simulink model "LPDs_single_agent_tech"  (R2023b)
settings: Solver=VariableStepAuto  StartTime=0.0  StopTime=24  FixedStep=0.005  RelTol=1e-6
undefined symbols (not defined in the file): battery_capacity_state_lower_limit, battery_capacity_state_upper_limit, battery_charge_power_state_lower_limit, battery_charge_power_state_upper_limit, battery_discharge_power_state_lower_limit, battery_discharge_power_state_upper_limit, battery_initial_capacity, battery_SOC_state_lower_limit, battery_SOC_state_upper_limit, EV_load_priority_factor, EV_load_rating, EV_load_state_lower_limit, EV_load_state_upper_limit, micro_grid_controller_power_state_lower_limit, micro_grid_controller_power_state_upper_limit, nano_grid_controller_power_rating, nano_grid_controller_power_state_lower_limit, nano_grid_controller_power_state_upper_limit, PV_power_rating, PV_power_state_lower_limit, PV_power_state_upper_limit, static_load_priority_factor, static_load_rating, static_load_state_lower_limit, static_load_state_upper_limit, sum_power_threshold_lower_limit, sum_power_threshold_upper_limit, TCL_load_priority_factor, TCL_load_rating, TCL_load_state_lower_limit, TCL_load_state_upper_limit, Wind_power_rating, Wind_power_state_lower_limit, Wind_power_state_upper_limit
libraries: spsStairGeneratorLib x13, simulink x7, slpidlib x2, rllib x2
(part 2 of 4)

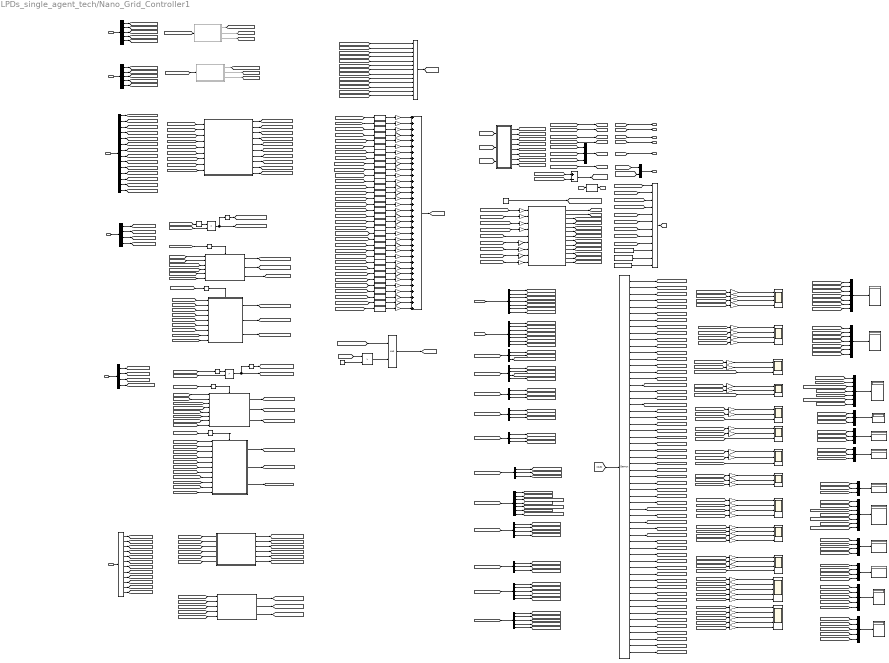
== system LPDs_single_agent_tech/Nano_Grid_Controller1 ==
  note: PV
  note: don't need I think so lets see it latter ???????????
  note: microgrid is least source
  note: nano grid is least priority source, its power usage will be punished:
      | if nanogrid is forecasting power supply
      | if nano grid is forecasting power consumption OR
      | if PV is NOT fully utilized OR
      | if wind is NOT fully utilized
  note: +ve = supply power
      | -ve = consume power
  note: Controller receiving
      | Information
      | ------------------------->
  note: Controller Transmitting
      | Information
  note: PV Power System parameters
      | ----------------------------------------------------------------------------------
  note: Wind
  note: BESS
  note: Load
  note: Observations / States / inputs
  note: Rewards / Punishments
  note: Battery is full and charging
      | than punish
  note: Micro Grid
  note: Nano Grid
  note: Wind Power System parameters
      | ----------------------------------------------------------------------------------
  note: Battery Power System parameters
      | ----------------------------------------------------------------------------------
  note: Nano Grid parameters
      | ----------------------------------------------------------------------------------
  note: Micro grid parameters
      | ----------------------------------------------------------------------------------
  note: Load parameters
      | ----------------------------------------------------------------------------------
  note: Power balance
      | ----------------------------------------------------------------------------------
  note: Nano Grid as source
      | ----------------------------------------------------------------------------------
  note: punish only if resources are not fully utilized
      | -10 points
  note: punish only if resources are not fully utilized
      | -10 points
  note: Battery Power -----> Battery Capacity (kWh) -----> Battery SOC Battery Charge Power
      | Battery Discharge Power
  PV1_input : Inport
  Wind_input : Inport  Port=2
  MG_Input : Inport  Port=3
  BESS_Input : Inport  Port=4
  Load_Input : Inport  Port=5
  NGC2_input : Inport  Port=6
  Abs1 : Abs  SaturateOnIntegerOverflow=off
  Abs2 : Abs  SaturateOnIntegerOverflow=off
  BESS : Subsystem
  Chart : Stateflow chart  TreatAsAtomicUnit=on
      settings: PortSchema="{\"entries\":[{\"content\":{\"sides\":[{\"content\":{\"connectorIds\":[\"In9\",\"In6\",\"In7\",\"In8\",\"In5\",\"In1\",\"In2\",\"In3\",\"In4\"]},\"type\":\"ConnectorPlacement.EquallySpacedRectSide\",\"uuid\":\"f3048845-fd52-425a-ab3b-550a9eb5c4bb\"},{\"content\":{\"connectorIds\":[\"Out1\",\"Out2\",\"Out3\",\"Out4\",\"Out10\",\"Out5\",\"Out6\",\"Out7\",\"Out9\",\"Out8\",\"Out11\",\"Out13\",\"Out12\"],\"side\":\"RIGHT\"},\"type\":\"ConnectorPlacement.EquallySpacedRectSide\",\"uuid\":\"2d1173df-378c-4293-a498-92c6385b9f9f\"},{\"content\":{\"side\":\"TOP\"},\"type\":\"ConnectorPlacement.EquallySpacedRectSide\",\"uuid\":\"05862f1f-9d24-4b39-880b-c5be5c8acb5d\"}]},\"type\":\"ConnectorPlacement.EquallySpacedConnector\",\"uuid\":\"30ceb18a-58fc-4555-bcd7-9edbd3426fbd\"}],\"packageUris\":[\"http://schema.mathworks.com/mf0/Connector/R2020b\"],\"version\":\"1.0\"}"
  Constant : Constant  Value=50
  Constant18 : Constant  Value=TCL_load_priority_factor
  Constant19 : Constant  Value=EV_load_priority_factor
  Constant20 : Constant  Value=static_load_priority_factor
  Constant6 : Constant  Value=0.95
  Data Type Conversion{10,12,14..45} (34 alike) : DataTypeConversion  SaturateOnIntegerOverflow=off  RndMeth=Floor
  Demux : Demux  Outputs=58
  Demux{1..2,18..19} (4 alike) : Demux  Outputs=5
  Demux{9..10,12..14,17} (6 alike) : Demux  Outputs=3
  Demux{5..6,11,16} (4 alike) : Demux
  Demux15 : Demux  Outputs=7
  Demux3 : Demux  Outputs=14
  Demux4 : Demux  Outputs=12
  Demux7 : Demux  Outputs=7
  Demux8 : Demux  Outputs=7
  Display{1,3..5,9..15,17} (12 alike) : Display
      Display1 settings: Format=bank
      Display10 settings: Format=bank
      Display12 settings: Format=bank
      Display13 settings: Format=bank
      Display14 settings: Format=bank
      Display15 settings: Format=bank
      Display17 settings: Format=bank
      Display4 settings: Format=bank
      Display5 settings: Format=bank
  Gain{,3,5,16,21..24} (8 alike) : Gain  Gain=1e3
  Gain1 : Gain  Gain=-10
  Gain{12..14,53..91} (42 alike) : Gain  Gain=0.001
  Gain15 : Gain  Gain=-10
  Gain{17,37,39,45..47,51} (7 alike) : Gain  Gain=20
  Gain18 : Gain  Gain=500
  Gain19 : Gain  Gain=-10
  Gain20 : Gain  Gain=10
  Gain25 : Gain  Gain=10
  Gain26 : Gain  Gain=-15
  Gain{27,30..31,33} (4 alike) : Gain
  Gain{28,35,38,40,43..44,48..50} (9 alike) : Gain  Gain=-20
  Gain29 : Gain  Gain=15
  Gain32 : Gain  Gain=-15
  Gain34 : Gain  Gain=-15
  Gain{36,41..42,52} (4 alike) : Gain  Gain=0
  Load : Subsystem
  MATLAB Function : MATLAB Function  TreatAsAtomicUnit=on
  Micro Grid power Over Limit : RelationalOperator  Operator=>  OutDataTypeStr=boolean  RndMeth=Simplest  InputSameDT=off
  Micro grid as load : Subsystem
  Micro grid as source : Subsystem  TreatAsAtomicUnit=on
  Micro grid controller forecast power demad : simulink/Logic and Bit Operations/Compare To Zero  relop=<  OutDataTypeStr=boolean
  Micro grid controller forecast power supply : simulink/Logic and Bit Operations/Compare To Zero  relop=>  OutDataTypeStr=boolean
  Mux : Mux  Inputs=13
  Mux{1,5..6,8} (4 alike) : Mux  Inputs=7
  Mux{3,7,9..11} (5 alike) : Mux  Inputs=3
  Mux12 : Mux
  Mux13 : Mux
  Mux14 : Mux  Inputs=5
  Mux15 : Mux  Inputs=5
  Mux2 : Mux  Inputs=2
  Mux4 : Mux  Inputs=12
  NOT : Logic  Operator=NOT  IconShape=distinctive  AllPortsSameDT=off  OutDataTypeStr=boolean
  NOT2 : Logic  Operator=NOT  IconShape=distinctive  AllPortsSameDT=off  OutDataTypeStr=boolean
  Nano Grid power Over Limit : RelationalOperator  Operator=>  OutDataTypeStr=boolean  RndMeth=Simplest  InputSameDT=off
  Nano Grid power Over Limit1 : RelationalOperator  Operator=>  OutDataTypeStr=boolean  RndMeth=Simplest  InputSameDT=off
  PV-System : Subsystem  Commented=on
  Scope{6..11} (6 alike) : Scope  NumInputPorts=3
  Scope{4..5,12..14} (5 alike) : Scope  NumInputPorts=4
  Scope15 : Scope  NumInputPorts=5
  Scope16 : Scope  NumInputPorts=5
  Subsystem1 : Subsystem
  Subsystem2 : Subsystem
  Sum : Sum  Inputs=+-
  Sum6 : Sum  Inputs=++++++++++++++++++++++++++++++++++
  Wind power utilization : Subsystem  Commented=on
  nano grid power utilization : Logic  IconShape=distinctive  AllPortsSameDT=off  OutDataTypeStr=boolean
  nano grid as load : Subsystem
  nano grid as source : Subsystem  TreatAsAtomicUnit=on
  nano grid controller forecast power demad : simulink/Logic and Bit Operations/Compare To Zero  relop=<  OutDataTypeStr=boolean
  nano grid controller forecast power supply : simulink/Logic and Bit Operations/Compare To Zero  relop=>  OutDataTypeStr=boolean
  NGC2_output : Outport
  BESS_Output : Outport  Port=2
  Load_Output : Outport  Port=3
  MG_Output : Outport  Port=4
  PV_Output : Outport  Port=5
  Wind_Output : Outport  Port=6
  wires:
  Wind_input/1 -> Demux2/1
  BESS_Input/1 -> Demux3/1
  PV1_input/1 -> Demux1/1
  [nano_grid_controller_action] -> [NGC2_output]  "nano grid power"
  Mux3/1 -> [Load_Output]
  Demux2/1 -> [wind_power_upper_limit]
  Demux2/2 -> [wind_power_lower_limit]
  Demux2/5 -> [wind_power_action_]
  Demux2/4 -> [wind_power_forecast]
  Demux1/1 -> [PV1_power_upper_limit]
  Demux1/4 -> [PV1_power_forecast]
  Demux1/5 -> [PV1_power_action_]
  Demux1/2 -> [PV1_power_lower_limit]
  Demux3/1 -> [battery_capacity_upper_limit]
  Demux3/3 -> [battery_capacity]
  Demux3/4 -> [battery_SOC_upper_limit]
  Demux3/2 -> [battery_capacity_lower_limit]
  Demux3/5 -> [battery_SOC_lower_limit]
  Demux3/6 -> [battery_SOC]
  Demux4/2 -> [static_load_lower_limit]
  Demux4/5 -> [TCL_load_upper_limit]
  Demux4/7 -> [TCL_load]
  Demux4/1 -> [static_load_upper_limit]
  Demux4/3 -> [static_load]
  Load_Input/1 -> Demux4/1
  Demux4/6 -> [TCL_load_lower_limit]
  Demux4/9 -> [EV_load_upper_limit]
  Demux4/10 -> [EV_load_lower_limit]
  Demux4/11 -> [EV_load]
  Demux1/3 -> [PV1_power]
  Demux2/3 -> [wind_power]
  Demux3/9 -> [battery_charging_power]
  Demux3/8 -> [battery_charging_power_lower_limit]
  Demux3/7 -> [battery_charging_power_upper_limit]
  Demux3/10 -> [battery_discharging_power_upper_limit]
  Demux3/11 -> [battery_discharging_power_lower_limit]
  Demux3/12 -> [battery_discharging_power]
  Demux5/3 -> [MG_power]
  Demux5/2 -> [MG_power_lower_limit]
  Demux5/1 -> [MG_power_upper_limit]
  MG_Input/1 -> Demux5/1
  Demux6/1 -> [Nano_grid_power_upper_limit]
  Demux6/3 -> [Nano_grid_power]
  Demux6/2 -> [Nano_grid_power_lower_limit]
  NGC2_input/1 -> Demux6/1
  Nano Grid power Over Limit/1 -> NOT/1, [Nano_grid_power_Punish]  "Nano Grid power Over Limit"
  [Nano_grid_power_upper_limit] -> Nano Grid power Over Limit/2
  [Nano_grid_power] -> Abs1/1
  Abs1/1 -> Nano Grid power Over Limit/1
  Abs2/1 -> Micro Grid power Over Limit/1
  [MG_power] -> Abs2/1
  [MG_power_upper_limit] -> Micro Grid power Over Limit/2
  Micro Grid power Over Limit/1 -> NOT2/1, [MG_power_Punish]  "Nano Grid power Over Limit"
  [Power_balance_Reward] -> nano grid power utilization/1
  [Static_Loads_action] -> Mux3/1
  [TCL_Loads_action] -> Mux3/2
  [EV_Loads_action] -> Mux3/3
  Demux4/4 -> [static_load_action]
  Demux4/8 -> [TCL_load_action]
  Demux4/12 -> [EV_load_action]
  [PV_Reward] -> nano grid as source/1(PV_Reward)
  [wind_Reward] -> nano grid as source/2(wind_Reward)
  [NGC2_output] -> NGC2_output/1
  Demux6/4 -> [nano_grid_controllers_action]
  nano grid as source/3(nano_grid_controllers_action_) -> [nano_grid_power_source]
  [MG_Output] -> MG_Output/1
  [Nano_grid_power] -> nano grid controller forecast power supply/1
  [nano_grid_controllers_action] -> nano grid as source/5(nano_grid_controllers_action)
  [Nano_grid_power] -> nano grid as source/6(nano_grid_controllers_power_supply)
  nano grid as source/2(Nano_grid_source_Punish) -> [Nano_grid_source_Punish]
  nano grid as source/1(Nano_grid_source_Reward) -> [Nano_grid_source_reward]
  [battery_capacity] -> BESS/1(battery_capacity)
  [battery_capacity_upper_limit] -> BESS/2(battery_capacity_upper_limit)
  [battery_SOC] -> BESS/3(battery_SOC)
  [battery_SOC_lower_limit] -> BESS/4(battery_SOC_lower_limit)
  [battery_discharging_power] -> BESS/8(battery_discharging_power)
  [battery_SOC_upper_limit] -> BESS/5(battery_SOC_upper_limit)
  [battery_charging_power] -> BESS/6(battery_charging_power)
  [battery_charging_power_upper_limit] -> BESS/7(battery_charging_power_upper_limit)
  [battery_discharging_power_upper_limit] -> BESS/9(battery_discharging_power_upper_limit)
  BESS/2(Battery capacity Punishment) -> [Battery_capacity_Punishment]
  BESS/4(Discharging at Low Battery SOC Punish) -> [discharge_Low_Battery_SOC_Punish]
  BESS/6(Overcharging Punish) -> [Battery_overcharging_Punish]
  BESS/8(Overcharging Rate Punish) -> [Battery_overcharging_rate_Punish]
  BESS/10(Overdischarging Rate Punish) -> [Battery_overdischarging_rate_Punish]
  [battery_discharging_power] -> nano grid as source/3(battery_discharging_power)
  [battery_discharging_power_upper_limit] -> nano grid as source/4(battery_discharging_power_upper_limit)
  [static_load_action] -> nano grid as load/1(static_load_action)
  [static_load] -> nano grid as load/2(static_load)
  [TCL_load_action] -> nano grid as load/3(TCL_load_action)
  [TCL_load] -> nano grid as load/4(TCL_load)
  [EV_load_action] -> nano grid as load/5(EV_load_action)
  [EV_load] -> nano grid as load/6(EV_load)
  [battery_SOC] -> nano grid as load/7(Battery_SOC)
  nano grid controller forecast power supply/1 -> nano grid as source/Enable
  [Nano_grid_power] -> nano grid controller forecast power demad/1
  nano grid controller forecast power demad/1 -> nano grid as load/Enable
  Wind power utilization/2(Wind_Reward) -> [wind_Reward]
  [Nano_grid_power] -> nano grid as load/9(nano_grid_controllers_power_demand)
  [nano_grid_controllers_action] -> nano grid as load/8(nano_grid_controllers_action)
  nano grid as load/2(Nano_grid_load_Punish) -> [Nano_grid_load_Punish]
  nano grid as load/3(nano_grid_controllers_action_) -> [nano_grid_load]
  nano grid as load/1(Nano_grid_load_Reward) -> [Nano_grid_load_reward]
  Micro grid as load/3(Micro_grid_controllers_action_) -> [micro_grid_load]
  Micro grid as load/1(Nano_grid_load_Reward) -> [micro_grid_load_reward]
  [Nano_grid_power] -> Micro grid as load/9(nano_grid_controllers_power_demand)
  Micro grid as load/2(Nano_grid_load_Punish) -> [micro_grid_load_Punish]
  Micro grid controller forecast power supply/1 -> Micro grid as source/Enable
  Micro grid as source/3(micro_grid_controllers_action_) -> [Micro_grid_power_source]
  [TCL_load] -> Micro grid as load/4(TCL_load)
  Micro grid controller forecast power demad/1 -> Micro grid as load/Enable
  [nano_grid_controllers_action] -> Micro grid as source/5(nano_grid_controllers_action)
  [PV_Reward] -> Micro grid as source/1(PV_Reward)
  [MG_power] -> Micro grid controller forecast power demad/1
  Micro grid as source/1(micro_grid_source_Reward) -> [Micro_grid_source_reward]
  [battery_SOC] -> Micro grid as load/7(Battery_SOC)
  [EV_load] -> Micro grid as load/6(EV_load)
  [battery_discharging_power_upper_limit] -> Micro grid as source/4(battery_discharging_power_upper_limit)
  [nano_grid_controllers_action] -> Micro grid as load/8(nano_grid_controllers_action)
  Micro grid as source/2(micro_grid_source_Punish) -> [Micro_grid_source_Punish]
  [battery_discharging_power] -> Micro grid as source/3(battery_discharging_power)
  [TCL_load_action] -> Micro grid as load/3(TCL_load_action)
  [Nano_grid_power] -> Micro grid as source/6(nano_grid_controllers_power_supply)
  [EV_load_action] -> Micro grid as load/5(EV_load_action)
  [static_load_action] -> Micro grid as load/1(static_load_action)
  [wind_Reward] -> Micro grid as source/2(wind_Reward)
  [static_load] -> Micro grid as load/2(static_load)
  [MG_power] -> Micro grid controller forecast power supply/1
  [micro_grid_controller_action] -> [MG_Output]  "micro grid power"
  Demux5/4 -> [micro_grid_controllers_action]
  [micro_grid_controllers_action] -> Micro grid as source/7(micro_grid_controllers_action)
  [MG_power] -> Micro grid as source/8(micro_grid_controllers_power_supply)
  [micro_grid_controllers_action] -> Micro grid as load/10(micro_grid_controllers_action)
  [MG_power] -> Micro grid as load/11(micro_grid_controllers_power_demand)
  Wind power utilization/3(Wind_punish) -> [wind_Punish]
  [PV_Output] -> PV_Output/1
  [PV_power_actions] -> [PV_Output]  "PV power command"
  [wind_power_actions] -> [Wind_Output]  "Wind power command"
  [Wind_Output] -> Wind_Output/1
  [wind_power] -> Wind power utilization/1(Wind_power)
  [Load_Output] -> Load_Output/1
  [static_load_action] -> Load/1(static_load_action)
  [static_load] -> Load/2(static_load)
  [TCL_load_action] -> Load/3(TCL_load_action)
  [TCL_load] -> Load/4(TCL_load)
  [EV_load_action] -> Load/5(EV_load_action)
  [EV_load] -> Load/6(EV_load)
  Load/1(static_load_reward) -> [static_load_reward]
  Load/2(static_load_punish) -> [static_load_punish]
  Load/3(TCL_load_reward) -> [TCL_load_reward]
  Load/4(TCL_load_punish) -> [TCL_load_punish]
  Load/5(EV_load_reward) -> [EV_load_reward]
  Load/6(EV_load_punish) -> [EV_load_punish]
  BESS/9(Overdischarging Rate Reward) -> [Battery_overdischarging_rate_Reward]
  BESS/7(Overcharging Rate Reward) -> [Battery_overcharging_rate_Reward]
  BESS/5(Overcharging Reward) -> [Battery_overcharging_Reward]
  BESS/3(Discharging at Low Battery SOC Reward) -> [discharge_Low_Battery_SOC_Reward]
  BESS/1(Battery capacity Reward) -> [Battery_capacity_Reward]
  NOT/1 -> [Nano_grid_power_Reward]
  NOT2/1 -> [MG_power_Reward]
  [PV1_power_action] -> Subsystem2/1(PV1_power_action)
  [wind_power_action] -> Subsystem2/2(wind_power_action)
  [static_load_action] -> Subsystem2/3(static_load_action)
  [TCL_load_action] -> Subsystem2/4(TCL_load_action)
  [EV_load_action] -> Subsystem2/5(EV_load_action)
  Subsystem2/1(Power_balance_Reward) -> [Power_balance_Reward]
  Subsystem2/2(Power_unbalance_Punish) -> [Power_unbalance_Punish]
  Subsystem2/3(Sum of powers) -> [sum_of_powers]
  [Rewards] -> Nano Grid power Over Limit1/1
  Constant/1 -> Nano Grid power Over Limit1/2
  Nano Grid power Over Limit1/1 -> nano grid power utilization/2  "Nano Grid power Over Limit"
  nano grid power utilization/1 -> [Isdone]
  [PV1_power] -> PV-System/1(PV1_power)
  PV-System/2(PV_Reward) -> [PV_Reward]
  PV-System/3(PV_punish) -> [PV_punish]
  PV-System/1(PV1_power_actions) -> [PV_power_action]
  Wind power utilization/1(Wind_power_actions) -> [wind_power_action]
  [wind_power] -> Gain3/1
  [Nano_grid_power] -> Gain21/1
  [TCL_load] -> Gain23/1
  [EV_load] -> Gain24/1
  [static_load] -> Gain22/1
  [BESS_action] -> [BESS_Output]  "charging or discharging power"
  Chart/1(PV_param) -> [PV_param]
  Chart/2(wind_param) -> [wind_param]
  Chart/3(battery_discharging_param) -> [battery_discharging_param]
  Chart/4(battery_charging_param) -> [battery_charging_param]
  Chart/5(static_load_param) -> [static_load_param]
  Chart/6(TCL_load_param) -> [TCL_load_param]
  Chart/7(EV_load_param) -> [EV_load_param]
  Chart/8(nano_grid_demand_param) -> [nano_grid_demand_param]
  Chart/9(nano_grid_supply_param) -> [nano_grid_supply_param]
  Chart/10(mg_param) -> [mg_param]
  Chart/11(load_source_balance) -> [load_source_balance]
  [PV_param] -> Demux7/1
  Demux7/1 -> [PV1_powers1]
  Demux7/2 -> [PV_load_usage1]
  Demux7/3 -> [PV_nanogrid_usage1]
  Demux7/4 -> [PV_remain_1]
  Demux7/5 -> [PV_load_usage_percentage1]
  Demux7/6 -> [PV_nanogrid_usage_percentage1]
  [wind_param] -> Demux8/1
  Demux9/3 -> [battery_charging_power_out_percentage1]
  [battery_charging_param] -> Demux9/1
  Demux9/1 -> [battery_charging_powers1]
  Demux9/2 -> [battery_charging_power_out1]
  Demux10/3 -> [static_load_usage_percentage1]
  Demux10/2 -> [static_load_usage1]
  Demux10/1 -> [static_loads1]
  [static_load_param] -> Demux10/1
  Demux11/3 -> [battery_discharging_power_out_percentage1]
  [battery_discharging_param] -> Demux11/1
  Demux11/2 -> [battery_discharging_power_out1]
  Demux11/1 -> [battery_discharging_powers1]
  Demux12/2 -> [TCL_load_usage1]
  Demux12/1 -> [TCL_loads1]
  [TCL_load_param] -> Demux12/1
  Demux12/3 -> [TCL_load_usage_percentage1]
  Demux13/2 -> [EV_load_usage1]
  Demux13/1 -> [EV_loads1]
  Demux13/3 -> [EV_load_usage_percentage1]
  [EV_load_param] -> Demux13/1
  [nano_grid_supply_param] -> Demux14/1
  Demux14/3 -> [nano_grid_remain1]
  Demux14/1 -> [nano_grid_supply1]
  Demux14/2 -> [nano_grid_usage1]
  Demux15/1 -> [nano_grid_demand1]
  Demux15/3 -> [nano_grid_demand_PV_usage_percentage1]
  Demux15/5 -> [nano_grid_demand_wind_usage_percentage1]
  Demux15/2 -> [nano_grid_demand_PV_usages1]
  Demux15/4 -> [nano_grid_demand_wind_usages1]
  Demux15/6 -> [nano_grid_demand_mg_usage1]
  [nano_grid_demand_param] -> Demux15/1
  Demux15/7 -> [nano_grid_demand_mg_usage_percentage1]
  Demux16/4 -> [mg_power_usage_nanogrid1]
  Demux16/2 -> [mg_power_usage1]
  Demux16/3 -> [mg_power_usage_load1]
  [mg_param] -> Demux16/1
  Demux17/2 -> [total_power_consumed1]
  Demux17/1 -> [total_power_produced1]
  Demux17/3 -> [power_balance_error1]
  [load_source_balance] -> Demux17/1
  Demux7/7 -> [PV_remain_percentage1]
  Demux8/6 -> [wind_nanogrid_usage_percentage1]
  Demux8/2 -> [wind_load_usage1]
  Demux8/7 -> [wind_remain_percentage1]
  Demux8/4 -> [wind_remain_1]
  Demux8/5 -> [wind_load_usage_percentage1]
  Demux8/1 -> [wind_powers1]
  Demux8/3 -> [wind_nanogrid_usage1]
  Gain/1 -> Chart/9(PV1_power)
  Gain3/1 -> Chart/6(wind_power)
  Gain5/1 -> Chart/7(battery_discharging_power)
  Gain16/1 -> Chart/8(battery_charging_power)
  Gain21/1 -> Chart/1(Nano_grid_power)
  Gain22/1 -> Chart/2(static_load)
  Gain23/1 -> Chart/3(TCL_load)
  Gain24/1 -> Chart/4(EV_load)
  Demux11/4 -> [battery_usage1]
  [PV1_power] -> Gain/1
  Demux3/13 -> [battery_charging_power_capacity]
  Demux3/14 -> [battery_discharging_power_capacity]
  [battery_charging_power_out] -> Sum/1
  [battery_discharging_power_out] -> Sum/2
  Sum/1 -> [battery_power]
  Mux2/1 -> BESS_Output/1
  [battery_power] -> Mux2/1
  [initial_battery_SOC] -> Mux2/2
  Constant6/1 -> [initial_battery_SOC]
  Chart/12(power_consumption) -> [power_consumption]
  Chart/13(power_production) -> [power_production]
  Demux18/1 -> [PV1_power_1]
  [power_production] -> Demux18/1
  Demux18/5 -> [mg_power_usage_1]
  Demux18/2 -> [wind_power_1]
  Demux18/3 -> [battery_discharging_power__1]
  Demux18/4 -> [nano_grid_supply_1]
  Demux19/3 -> [EV_load_usage_1]
  Demux19/1 -> [static_load_usage_1]
  Demux19/4 -> [battery_charging_power_out_1]
  Demux19/2 -> [TCL_load_usage_1]
  Demux19/5 -> [nano_grid_demand_1]
  [power_consumption] -> Demux19/1
  [PV1_powers] -> Gain12/1
  [PV_load_usage] -> Gain13/1
  [PV_nanogrid_usage] -> Gain14/1
  [PV_remain_] -> Gain53/1
  [wind_powers] -> Gain54/1
  [wind_load_usage] -> Gain55/1
  [wind_nanogrid_usage] -> Gain56/1
  [wind_remain_] -> Gain57/1
  [battery_charging_power_out] -> Gain59/1
  [battery_charging_powers] -> Gain58/1
  [battery_discharging_powers] -> Gain60/1
  [battery_discharging_power_out] -> Gain61/1
  [battery_discharging_power_out_percentage] -> Scope7/3  "battery_discharging_power_out_percentage"
  [static_loads] -> Gain62/1
  [static_load_usage] -> Gain63/1
  [TCL_load_usage] -> Gain65/1
  [TCL_loads] -> Gain64/1
  [EV_loads] -> Gain66/1
  [EV_load_usage] -> Gain67/1
  [nano_grid_supply] -> Gain68/1
  [nano_grid_usage] -> Gain69/1
  [nano_grid_remain] -> Gain70/1
  [mg_power_usage] -> Gain76/1
  [mg_power_usage_load] -> Gain77/1
  [mg_power_usage_nanogrid] -> Gain78/1
  [total_power_produced] -> Gain79/1
  [total_power_consumed] -> Gain80/1
  [power_balance_error] -> Gain81/1
  [nano_grid_demand] -> Gain71/1
  [nano_grid_demand_PV_usages] -> Gain72/1
  [nano_grid_demand_wind_usages] -> Gain73/1
  [nano_grid_demand_mg_usage] -> Gain74/1
  [PV1_power_] -> Gain82/1
  [wind_power_] -> Gain83/1
  [battery_discharging_power__] -> Gain84/1
  [nano_grid_supply_] -> Gain85/1
  [mg_power_usage_] -> Gain86/1
  [static_load_usage_] -> Gain87/1
  [TCL_load_usage_] -> Gain88/1
  [EV_load_usage_] -> Gain89/1
  [battery_charging_power_out_] -> Gain90/1
  [nano_grid_demand_] -> Gain91/1
  Data Type Conversion23/1 -> Gain1/1
  [Nano_grid_load_reward] -> Data Type Conversion33/1
  Data Type Conversion41/1 -> Gain47/1
  Data Type Conversion43/1 -> Gain49/1
  [static_load_reward] -> Data Type Conversion41/1
  Gain44/1 -> Sum6/24
  Data Type Conversion42/1 -> Gain48/1
  [Battery_overdischarging_rate_Reward] -> Data Type Conversion28/1
  [TCL_load_reward] -> Data Type Conversion40/1
  Gain48/1 -> Sum6/28
  [MG_power_Reward] -> Data Type Conversion35/1
  [micro_grid_load_Punish] -> Data Type Conversion37/1
  [Micro_grid_source_reward] -> Data Type Conversion20/1
  Gain49/1 -> Sum6/32
  [Power_balance_Reward] -> Data Type Conversion21/1
  Gain47/1 -> Sum6/27
  [PV_Reward] -> Data Type Conversion14/1
  Gain37/1 -> Sum6/17
  [micro_grid_load_reward] -> Data Type Conversion39/1
  Gain50/1 -> Sum6/30
  [Nano_grid_load_Punish] -> Data Type Conversion34/1
  Gain43/1 -> Sum6/26
  Data Type Conversion32/1 -> Gain38/1
  Data Type Conversion30/1 -> Gain36/1
  [battery_discharging_power] -> Mux/8
  Gain15/1 -> Sum6/4
  Gain26/1 -> Sum6/6
  Gain34/1 -> Sum6/14
  [EV_load_punish] -> Data Type Conversion43/1
  [static_load_punish] -> Data Type Conversion42/1
  Gain20/1 -> Sum6/1
  [wind_power_forecast] -> Mux/4
  Data Type Conversion45/1 -> Gain51/1
  Gain51/1 -> Sum6/31
  [Nano_grid_power_Reward] -> Data Type Conversion19/1
  Gain46/1 -> Sum6/29
  Gain35/1 -> Sum6/10
  Gain45/1 -> Sum6/25
  Gain1/1 -> Sum6/2
  Gain38/1 -> Sum6/18
  Gain33/1 -> Sum6/13
  Data Type Conversion24/1 -> Gain15/1
  Gain41/1 -> Sum6/21
  [discharge_Low_Battery_SOC_Reward] -> Data Type Conversion15/1
  [EV_load_reward] -> Data Type Conversion45/1
  Data Type Conversion26/1 -> Gain31/1
  [Nano_grid_power_Punish] -> Data Type Conversion30/1
  Data Type Conversion29/1 -> Gain34/1
  Data Type Conversion40/1 -> Gain46/1
  Data Type Conversion25/1 -> Gain30/1
  Gain19/1 -> Sum6/34
  Gain29/1 -> Sum6/9
  [Micro_grid_source_Punish] -> Data Type Conversion38/1
  Gain18/1 -> Sum6/33
  Data Type Conversion22/1 -> Gain19/1
  [wind_Reward] -> Data Type Conversion12/1
  [TCL_load] -> Mux/12
  [MG_power] -> Mux/10
  [battery_charging_power] -> Mux/7
  [Battery_capacity_Punishment] -> Data Type Conversion10/1
  Data Type Conversion21/1 -> Gain18/1
  [battery_capacity] -> Mux/5
  Data Type Conversion36/1 -> Gain42/1
  [Battery_overdischarging_rate_Punish] -> Data Type Conversion29/1
  Sum6/1 -> [Rewards]
  Data Type Conversion38/1 -> Gain44/1
  Gain31/1 -> Sum6/11
  Gain42/1 -> Sum6/22
  [Nano_grid_source_Punish] -> Data Type Conversion32/1
  Gain40/1 -> Sum6/20
  Data Type Conversion14/1 -> Gain20/1
  Gain17/1 -> Sum6/23
  Data Type Conversion16/1 -> Gain28/1
  [Battery_overcharging_rate_Reward] -> Data Type Conversion26/1
  Data Type Conversion20/1 -> Gain17/1
  Data Type Conversion28/1 -> Gain33/1
  Gain39/1 -> Sum6/19
  Data Type Conversion34/1 -> Gain40/1
  Data Type Conversion31/1 -> Gain37/1
  Gain36/1 -> Sum6/16
  [Nano_grid_power] -> Mux/9
  [PV1_power_forecast] -> Mux/2
  Gain32/1 -> Sum6/12
  [EV_load] -> Mux/13
  [Battery_overcharging_Punish] -> Data Type Conversion18/1
  Data Type Conversion17/1 -> Gain29/1
  [Battery_overcharging_Reward] -> Data Type Conversion17/1
  Data Type Conversion44/1 -> Gain50/1
  Data Type Conversion27/1 -> Gain32/1
  [Nano_grid_source_reward] -> Data Type Conversion31/1
  [wind_Punish] -> Data Type Conversion24/1
  [Battery_overcharging_rate_Punish] -> Data Type Conversion27/1
  Data Type Conversion10/1 -> Gain26/1
  Gain28/1 -> Sum6/8
  Data Type Conversion39/1 -> Gain45/1
  Data Type Conversion33/1 -> Gain39/1
  [discharge_Low_Battery_SOC_Punish] -> Data Type Conversion16/1
  Data Type Conversion35/1 -> Gain41/1
  Gain30/1 -> Sum6/5
  [PV_punish] -> Data Type Conversion23/1
  [MG_power_Punish] -> Data Type Conversion36/1
  [Battery_capacity_Reward] -> Data Type Conversion25/1
  Gain27/1 -> Sum6/7
  [Power_unbalance_Punish] -> Data Type Conversion22/1
  Gain52/1 -> Sum6/15
  [static_load] -> Mux/11
  Gain25/1 -> Sum6/3
  Data Type Conversion15/1 -> Gain27/1
  [TCL_load_punish] -> Data Type Conversion44/1
  Data Type Conversion12/1 -> Gain25/1
  Data Type Conversion19/1 -> Gain52/1
  [PV1_power] -> Mux/1
  [battery_SOC] -> Mux/6
  Data Type Conversion18/1 -> Gain35/1
  Mux/1 -> [Observations]
  [wind_power] -> Mux/3
  Data Type Conversion37/1 -> Gain43/1
  [Isdone] -> Subsystem1/3(isdone)
  [Observations] -> Subsystem1/1(observation)
  [Rewards] -> Subsystem1/2(reward)
  Subsystem1/1(Out1) -> [PV_power_actions]
  Subsystem1/2(Out2) -> [wind_power_actions]
  Subsystem1/3(Out3) -> [BESS_action]
  Subsystem1/4(Out4) -> [nano_grid_controller_action]
  Subsystem1/5(Out5) -> [micro_grid_controller_action]
  Subsystem1/6(Out6) -> [Static_Loads_action]
  Subsystem1/7(Out7) -> [TCL_Loads_action]
  Subsystem1/8(Out8) -> [EV_Loads_action]
  [MG_power] -> Chart/5(micro_grid_power)
  Demux16/1 -> [mg_power1]
  [mg_power] -> Gain75/1
  Mux4/1 -> [input]
  MATLAB Function/1(y) -> [out]
  [EV_load] -> Mux4/9
  [TCL_load] -> Mux4/8
  [static_load] -> Mux4/7
  [Nano_grid_power] -> Mux4/6
  [wind_power] -> Mux4/2
  [battery_discharging_power_capacity] -> Mux4/3
  [battery_charging_power_capacity] -> Mux4/4
  Constant20/1 -> Mux4/10
  Constant18/1 -> Mux4/11
  Constant19/1 -> Mux4/12
  [MG_power] -> Mux4/5
  Demux/21 -> [battery_usage]
  Demux/6 -> [PV_nanogrid_usage_percentage]
  Demux/9 -> [wind_load_usage]
  Demux/13 -> [wind_nanogrid_usage_percentage]
  Demux/42 -> [mg_power_usage]
  Demux/53 -> [static_load_usage_]
  Demux/50 -> [battery_discharging_power__]
  Demux/54 -> [TCL_load_usage_]
  Demux/15 -> [battery_charging_powers]
  Demux/16 -> [battery_charging_power_out]
  Demux/49 -> [wind_power_]
  Demux/12 -> [wind_load_usage_percentage]
  Demux/31 -> [nano_grid_supply]
  Demux/34 -> [nano_grid_demand]
  Demux/30 -> [EV_load_usage_percentage]
  Demux/40 -> [nano_grid_demand_mg_usage_percentage]
  Demux/10 -> [wind_nanogrid_usage]
  Demux/26 -> [TCL_load_usage]
  Demux/48 -> [PV1_power_]
  Demux/41 -> [mg_power]
  Demux/23 -> [static_load_usage]
  Demux/24 -> [static_load_usage_percentage]
  Demux/25 -> [TCL_loads]
  Demux/18 -> [battery_discharging_powers]
  Demux/5 -> [PV_load_usage_percentage]
  Demux/45 -> [total_power_produced]
  Demux/4 -> [PV_remain_]
  Demux/47 -> [power_balance_error]
  Demux/35 -> [nano_grid_demand_PV_usages]
  Demux/36 -> [nano_grid_demand_PV_usage_percentage]
  Demux/32 -> [nano_grid_usage]
  Demux/33 -> [nano_grid_remain]
  Demux/28 -> [EV_loads]
  Demux/29 -> [EV_load_usage]
  Demux/27 -> [TCL_load_usage_percentage]
  Demux/44 -> [mg_power_usage_nanogrid]
  Demux/3 -> [PV_nanogrid_usage]
  Demux/14 -> [wind_remain_percentage]
  Demux/37 -> [nano_grid_demand_wind_usages]
  Demux/7 -> [PV_remain_percentage]
  Demux/22 -> [static_loads]
  Demux/51 -> [nano_grid_supply_]
  Demux/11 -> [wind_remain_]
  Demux/1 -> [PV1_powers]
  Demux/56 -> [battery_charging_power_out_]
  Demux/39 -> [nano_grid_demand_mg_usage]
  Demux/52 -> [mg_power_usage_]
  Demux/38 -> [nano_grid_demand_wind_usage_percentage]
  Demux/2 -> [PV_load_usage]
  Demux/55 -> [EV_load_usage_]
  Demux/46 -> [total_power_consumed]
  Demux/43 -> [mg_power_usage_load]
  Demux/19 -> [battery_discharging_power_out]
  Demux/57 -> [nano_grid_demand_]
  Demux/8 -> [wind_powers]
  [out] -> Demux/1
  Demux/17 -> [battery_charging_power_out_percentage]
  Demux/20 -> [battery_discharging_power_out_percentage]
  [PV1_powers] -> Mux1/1
  [PV_load_usage] -> Mux1/2
  [PV_nanogrid_usage] -> Mux1/3
  [PV_remain_] -> Mux1/4
  [PV_load_usage_percentage] -> Mux1/5
  [PV_nanogrid_usage_percentage] -> Mux1/6
  [PV_remain_percentage] -> Mux1/7
  Mux1/1 -> Display1/1
  [wind_load_usage] -> Mux5/2
  [wind_powers] -> Mux5/1
  [wind_nanogrid_usage] -> Mux5/3
  [wind_remain_] -> Mux5/4
  [wind_load_usage_percentage] -> Mux5/5
  [wind_nanogrid_usage_percentage] -> Mux5/6
  [wind_remain_percentage] -> Mux5/7
  Mux5/1 -> Display15/1
  [battery_charging_powers] -> Mux6/1
  [battery_charging_power_out] -> Mux6/2
  [battery_charging_power_out_percentage] -> Mux6/3
  [battery_discharging_powers] -> Mux6/4
  [battery_discharging_power_out] -> Mux6/5
  [battery_discharging_power_out_percentage] -> Mux6/6
  [battery_usage] -> Mux6/7
  Mux6/1 -> Display4/1
  [nano_grid_usage] -> Mux7/2
  [nano_grid_remain] -> Mux7/3
  [nano_grid_supply] -> Mux7/1
  Mux7/1 -> Display10/1
  [nano_grid_demand] -> Mux8/1
  [nano_grid_demand_PV_usages] -> Mux8/2
  [nano_grid_demand_PV_usage_percentage] -> Mux8/3
  [nano_grid_demand_wind_usages] -> Mux8/4
  Mux8/1 -> Display13/1
  [nano_grid_demand_wind_usage_percentage] -> Mux8/5
  [nano_grid_demand_mg_usage] -> Mux8/6
  [nano_grid_demand_mg_usage_percentage] -> Mux8/7
  [static_loads] -> Mux9/1
  [static_load_usage] -> Mux9/2
  [static_load_usage_percentage] -> Mux9/3
  Mux9/1 -> Display5/1
  [TCL_loads] -> Mux10/1
  [TCL_load_usage] -> Mux10/2
  [TCL_load_usage_percentage] -> Mux10/3
  Mux10/1 -> Display3/1
  [EV_loads] -> Mux11/1
  [EV_load_usage] -> Mux11/2
  [EV_load_usage_percentage] -> Mux11/3
  Mux11/1 -> Display9/1
  [mg_power] -> Mux12/1
  [mg_power_usage] -> Mux12/2
  [mg_power_usage_load] -> Mux12/3
  [mg_power_usage_nanogrid] -> Mux12/4
  Mux12/1 -> Display11/1
  [total_power_produced] -> Mux13/1
  [total_power_consumed] -> Mux13/2
  [power_balance_error] -> Mux13/3
  [PV1_power_] -> Mux14/1
  [wind_power_] -> Mux14/2
  [battery_discharging_power__] -> Mux14/3
  [nano_grid_supply_] -> Mux14/4
  [mg_power_usage_] -> Mux14/5
  Mux14/1 -> Display17/1
  [TCL_load_usage_] -> Mux15/2
  [EV_load_usage_] -> Mux15/3
  [battery_charging_power_out_] -> Mux15/4
  [nano_grid_demand_] -> Mux15/5
  [static_load_usage_] -> Mux15/1
  Mux13/1 -> Display12/1
  Mux15/1 -> Display14/1
  [static_load_usage_percentage] -> Scope8/3  "static_load_usage_percentage"
  [TCL_load_usage_percentage] -> Scope9/3  "TCL_load_usage_percentage"
  [EV_load_usage_percentage] -> Scope10/3  "EV_load_usage_percentage"
  [battery_charging_power_out_percentage] -> Scope6/3  "battery_charging_power_out_percentage"
  Gain13/1 -> Scope4/2  "PV_load_usage (kW)"
  Gain14/1 -> Scope4/3  "PV_nanogrid_usage (kW)"
  Gain53/1 -> Scope4/4  "PV_remain_ (kW)"
  Gain54/1 -> Scope5/1  "wind_powers (kW)"
  Gain55/1 -> Scope5/2  "wind_load_usage (kW)"
  Gain56/1 -> Scope5/3  "wind_nanogrid_usage (kW)"
  Gain57/1 -> Scope5/4  "wind_remain_ (kW)"
  Gain58/1 -> Scope6/1  "battery_charging_powers (kW)"
  Gain59/1 -> Scope6/2  "battery_charging_power_out (kW)"
  Gain60/1 -> Scope7/1  "battery_discharging_powers (kW)"
  Gain12/1 -> Scope4/1  "PV1_powers (kW)"
  Gain61/1 -> Scope7/2  "battery_discharging_power_out (kW)"
  Gain62/1 -> Scope8/1  "static_loads (kW)"
  Gain63/1 -> Scope8/2  "static_load_usage (kW)"
  Gain64/1 -> Scope9/1  "TCL_loads (kW)"
  Gain65/1 -> Scope9/2  "TCL_load_usage (kW)"
  Gain66/1 -> Scope10/1  "EV_loads (kW)"
  Gain67/1 -> Scope10/2  "EV_load_usage (kW)"
  Gain68/1 -> Scope11/1  "nano_grid_supply (kW)"
  Gain69/1 -> Scope11/2  "nano_grid_usage (kW)"
  Gain70/1 -> Scope11/3  "nano_grid_remain (kW)"
  Gain71/1 -> Scope14/1  "nano_grid_demand (kW)"
  Gain72/1 -> Scope14/2  "nano_grid_demand_PV_usages (kW)"
  Gain73/1 -> Scope14/3  "nano_grid_demand_wind_usages (kW)"
  Gain74/1 -> Scope14/4  "nano_grid_demand_mg_usage (kW)"
  Gain75/1 -> Scope12/1  "mg_power (kW)"
  Gain76/1 -> Scope12/2  "mg_power_usage (kW)"
  Gain77/1 -> Scope12/3  "mg_power_usage_load (kW)"
  Gain78/1 -> Scope12/4  "mg_power_usage_nanogrid (kW)"
  Gain80/1 -> Scope13/2  "total_power_consumed (kW)"
  Gain79/1 -> Scope13/1  "total_power_produced (kW)"
  Gain81/1 -> Scope13/3  "power_balance_error (kW)"
  Gain83/1 -> Scope15/2  "wind_power_ (kW)"
  Gain84/1 -> Scope15/3  "battery_discharging_power__ (kW)"
  Gain82/1 -> Scope15/1  "PV1_power_ (kW)"
  Gain85/1 -> Scope15/4  "nano_grid_supply_ (kW)"
  Gain86/1 -> Scope15/5  "mg_power_usage_ (kW)"
  Gain87/1 -> Scope16/1  "static_load_usage_ (kW)"
  Gain88/1 -> Scope16/2  "TCL_load_usage_ (kW)"
  Gain90/1 -> Scope16/4  "battery_charging_power_out_ (kW)"
  Gain89/1 -> Scope16/3  "EV_load_usage_ (kW)"
  Gain91/1 -> Scope16/5  "nano_grid_demand_ (kW)"
  [input] -> MATLAB Function/1(u)
  Demux/58 -> [error]
  [error] -> Scope13/4  "error"
  [error] -> Mux13/4  "error"
  [battery_discharging_power_capacity] -> Gain5/1
  [battery_charging_power_capacity] -> Gain16/1
  [PV1_power] -> Mux4/1

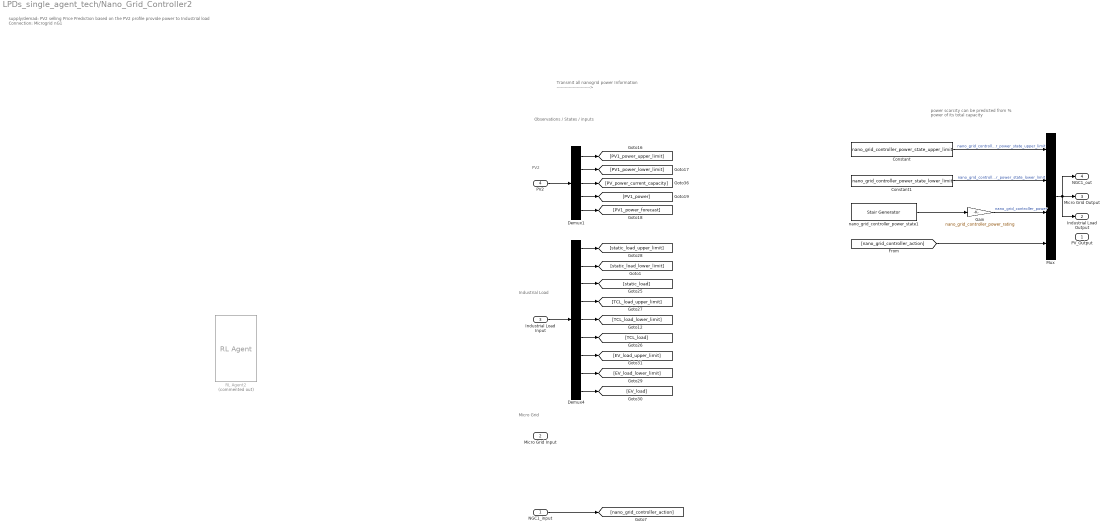
== system LPDs_single_agent_tech/Nano_Grid_Controller2 ==
  note: supply/demad:
      | PV2 selling Price Prediction based on the PV2 profile
      | provide power to Industrial load
      |
      | Connection:
      | Microgrid
      | nG1
  note: Transmit all nanogrid power Information
      | ------------------------->
  note: power scarcity can be predicted from % power of its total capacity
  note: PV2
  note: Observations / States / inputs
  note: Industrial
      | Load
  note: Micro Grid
  NGC1_input : Inport
  Micro Grid Input : Inport  Port=2
  Industrial Load Input : Inport  Port=3
  PV2 : Inport  Port=4
  Constant : Constant  Value=nano_grid_controller_power_state_upper_limit
  Constant1 : Constant  Value=nano_grid_controller_power_state_lower_limit
  Demux1 : Demux  Outputs=5
  Demux4 : Demux  Outputs=9
  Gain : Gain  Gain=nano_grid_controller_power_rating
  Mux : Mux
  RL Agent2 : rllib/RL Agent  Commented=on  Agent=agent1  ExternalActionAsInput=off  ProvideLastAction=off  ProvideCumRwd=off  TreatAsDirectFeedthrough=on  UseStrictObservationDataTypes=off
  nano_grid_controller_power_state1 : spsStairGeneratorLib/Stair Generator  t=[0, 1, 2, 3, 4, 5, 6, 7, 8, 9, 10, 11, 12, 13, 14, 15, 16, 17, 18, 19, 20, 21, 22, 23]  e=[-0.8, -0.9, -1, -0.9, -0.8, -0.7, -0.6, -0.5, -0.4, -0.3, -0.2, -0.1, 0, 0.1, 0.2, 0.3, 0.4, 0.5, 0.6, 0.7, 0.8, 0.9, 1, 0]  Ts=0
  PV_Output : Outport
  Industrial Load Output : Outport  Port=2
  Micro Grid Output : Outport  Port=3
  NGC1_out : Outport  Port=4
  wires:
  Constant1/1 -> Mux/2  "nano_grid_controller_power_state_lower_limit"
  nano_grid_controller_power_state1/1 -> Gain/1
  Constant/1 -> Mux/1  "nano_grid_controller_power_state_upper_limit"
  Gain/1 -> Mux/3  "nano_grid_controller_power"
  Mux/1 -> Industrial Load Output/1, NGC1_out/1, Micro Grid Output/1
  Demux1/2 -> [PV1_power_lower_limit]
  Demux1/4 -> [PV1_power]
  PV2/1 -> Demux1/1
  Demux1/1 -> [PV1_power_upper_limit]
  Demux1/3 -> [PV_power_current_capacity]
  Demux1/5 -> [PV1_power_forecast]
  Demux4/1 -> [static_load_upper_limit]
  Demux4/3 -> [static_load]
  Demux4/9 -> [EV_load]
  Demux4/5 -> [TCL_load_lower_limit]
  Demux4/4 -> [TCL_load_upper_limit]
  Demux4/7 -> [EV_load_upper_limit]
  Demux4/6 -> [TCL_load]
  Demux4/8 -> [EV_load_lower_limit]
  Demux4/2 -> [static_load_lower_limit]
  Industrial Load Input/1 -> Demux4/1
  NGC1_input/1 -> [nano_grid_controller_action]
  [nano_grid_controller_action] -> Mux/4

== system LPDs_single_agent_tech/PV1_100kW ==
  note: Transmit all PV power Information
      | ------------------------->
  note: real time PV Power production based on solar irradiance
  PV_Output : Inport
  Constant : Constant  Value=PV_power_state_upper_limit
  Constant1 : Constant  Value=PV_power_state_lower_limit
  Gain : Gain  Gain=1/100
  Gain1 : Gain  Gain=PV_power_rating
  Gain2 : Gain  Gain=PV_power_rating
  Gain3 : Gain  Gain=1/100
  Mux1 : Mux  Inputs=5
  PV1_power_forecast : Constant  Value=100000
  PV1_power_forecast1 : spsStairGeneratorLib/Stair Generator  t=[0, 1, 2, 3, 4, 5, 6, 7, 8, 9, 10, 11, 12, 13, 14, 15, 16, 17, 18, 19, 20, 21, 22, 23]  e=[0, 0, 0, 0, 0, 0, 0, 12.5, 25, 37.5, 50, 62.5, 75, 87.5, 100, 87.5, 75, 62.5, 50, 37.5, 25, 12.5, 0, 0];  Ts=0
  PV1_power_state : Constant  Value=0.9
  PV1_power_state1 : spsStairGeneratorLib/Stair Generator  t=[0, 1, 2, 3, 4, 5, 6, 7, 8, 9, 10, 11, 12, 13, 14, 15, 16, 17, 18, 19, 20, 21, 22, 23]  e=[0, 0, 0, 0, 0, 0, 12.5, 25, 37.5, 50, 62.5, 75, 87.5, 100, 87.5, 75, 62.5, 50, 37.5, 25, 12.5, 0, 0, 0];  Ts=0
  Scope : Scope
  NGC1_output : Outport
  wires:
  Constant/1 -> Mux1/1  "PV1_upper_capacity"
  Mux1/1 -> NGC1_output/1
  Constant1/1 -> Mux1/2  "PV1_lower_capacity"
  PV1_power_forecast/1 -> ?
  Gain1/1 -> Mux1/4  "PV1_power_forecast"
  PV1_power_state/1 -> ?
  Gain2/1 -> Scope/1, Mux1/3  "PV1_power_state"
  [PV_Power_action] -> Mux1/5  "PV Power action feeding to the load  commanded by controller"
  PV_Output/1 -> [PV_Power_action]  "PV Power action feeding to the load  commanded by controller"
  PV1_power_state1/1 -> Gain/1
  PV1_power_forecast1/1 -> Gain3/1
  Gain/1 -> Gain2/1
  Gain3/1 -> Gain1/1

== system LPDs_single_agent_tech/PV2 (100 kW) ==
  note: Transmit all PV power Information
      | ------------------------->
  note: real time PV Power production based on solar irradiance
  PV_Output : Inport
  Constant : Constant  Value=PV_power_state_upper_limit
  Constant1 : Constant  Value=PV_power_state_lower_limit
  Gain : Gain
  Gain1 : Gain  Gain=PV_power_rating
  Gain2 : Gain  Gain=PV_power_rating
  Mux1 : Mux  Inputs=5
  Real time PV Power production based on solar irradiance : spsStairGeneratorLib/Stair Generator  t=[0, 1, 2, 3, 4, 5, 6, 7, 8, 9, 10, 11, 12, 13, 14, 15, 16, 17, 18, 19, 20, 21, 22, 23]  e=[0, 0, 0, 0.1, 0, 0, 0, 0.1, 0.3, 0.5, 0.6, 0.7, 0.8, 0.9, 1, 0.8, 0.6, 0.4, 0.2, 0, 0, 0, 0, 0]  Ts=0
  Stair Generator1 : spsStairGeneratorLib/Stair Generator  t=[0, 1, 2, 3, 4, 5, 6, 7, 8, 9, 10, 11, 12, 13, 14, 15, 16, 17, 18, 19, 20, 21, 22, 23]  e=[0, 0, 0, 0, 0, 0, 0, 0.1, 0.3, 0.5, 0.6, 0.7, 0.8, 0.9, 1, 0.8, 0.6, 0.4, 0.2, 0, 0, 0, 0, 0]  Ts=0
  NGC1_output : Outport
  wires:
  Constant/1 -> Mux1/1  "PV1_upper_capacity"
  Mux1/1 -> NGC1_output/1
  Constant1/1 -> Mux1/2  "PV1_lower_capacity"
  Stair Generator1/1 -> Gain1/1
  Gain1/1 -> Mux1/4  "PV1_power_forecast"
  Real time PV Power production based on solar irradiance/1 -> Gain2/1
  Gain2/1 -> Mux1/3  "PV1_power_state"
  Gain/1 -> Mux1/5  "PV1_power_action"
  [PV_Power_action] -> Gain/1  "PV Power action feeding to the load  commanded by controller"
  PV_Output/1 -> [PV_Power_action]  "PV Power action feeding to the load  commanded by controller"

== system LPDs_single_agent_tech/Wind_20kW ==
  note: Transmit all Wind power Information
      | ------------------------->
  note: power scarcity can be predicted from % power of its total capacity
  Wind_Output : Inport
  Constant : Constant  Value=Wind_power_state_upper_limit
  Constant1 : Constant  Value=Wind_power_state_lower_limit
  Gain : Gain  Gain=Wind_power_rating
  Gain1 : Gain  Gain=Wind_power_rating
  Gain2 : Gain
  Gain3 : Gain  Gain=1/100
  Gain4 : Gain  Gain=1/100
  Mux : Mux  Inputs=5
  Wind_power_forecast : Constant  Value=100000
  Wind_power_forecast1 : spsStairGeneratorLib/Stair Generator  t=[0, 1, 2, 3, 4, 5, 6, 7, 8, 9, 10, 11, 12, 13, 14, 15, 16, 17, 18, 19, 20, 21, 22, 23]  e=[0, 0, 0, 25, 50, 75, 100, 80, 60, 40, 20, 0, 0, 0, 0, 0, 0, 0, 0, 0, 0, 0, 0, 0];  Ts=0
  Wind_power_state : Constant  Value=0.9
  Wind_power_state1 : spsStairGeneratorLib/Stair Generator  t=[0, 1, 2, 3, 4, 5, 6, 7, 8, 9, 10, 11, 12, 13, 14, 15, 16, 17, 18, 19, 20, 21, 22, 23]  e=[0, 0, 25, 50, 75, 100, 80, 60, 40, 20, 0, 0, 0, 0, 0, 0, 0, 0, 0, 0, 0, 0, 0, 0];  Ts=0
  NGC1_output : Outport
  wires:
  Mux/1 -> NGC1_output/1
  Constant/1 -> Mux/1  "wind_upper_capacity"
  Gain/1 -> Mux/4  "Wind_power_forecast"
  Constant1/1 -> Mux/2  "wind_lower_capacity"
  Wind_power_forecast1/1 -> Gain4/1
  Wind_power_state1/1 -> Gain3/1
  Wind_Output/1 -> [PV_Power_action]  "PV Power action feeding to the load  commanded by controller"
  [PV_Power_action] -> Gain2/1  "Wind Power action feeding to the load  commanded by controller"
  Gain2/1 -> Mux/5  "Wind_power_action"
  Gain1/1 -> Mux/3  "Wind_power_forecast"
  Gain3/1 -> Gain1/1
  Gain4/1 -> Gain/1

== system LPDs_single_agent_tech/BESS_10 kWh/Subsystem ==
  In1 : Inport
  Enable : EnablePort
  Out1 : Outport
  wires:
  In1/1 -> Out1/1

== system LPDs_single_agent_tech/BESS_10 kWh/Subsystem1 ==
  In1 : Inport
  Enable : EnablePort
  Out1 : Outport
  wires:
  In1/1 -> Out1/1

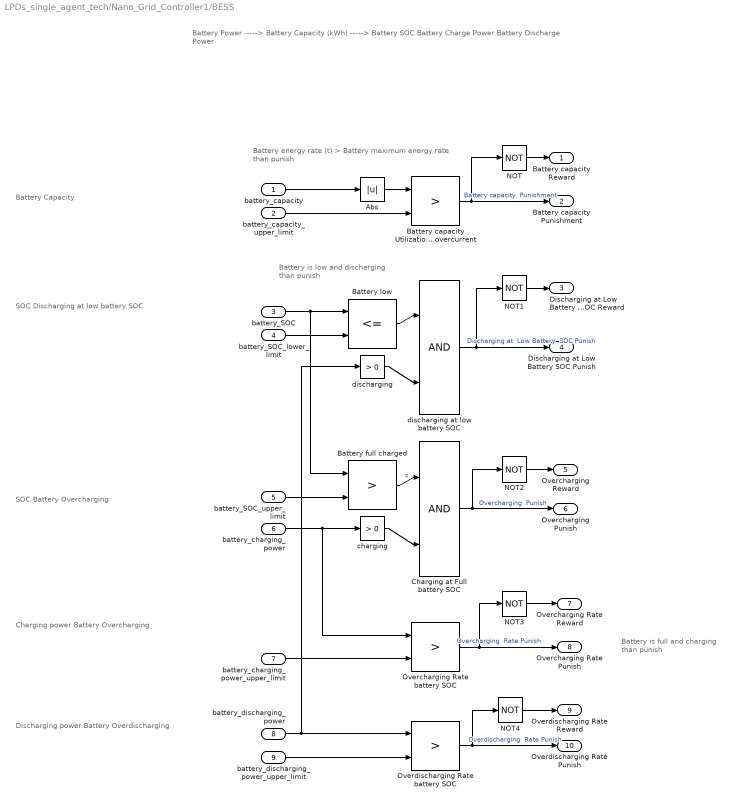
== system LPDs_single_agent_tech/Nano_Grid_Controller1/BESS ==
  note: Battery energy rate (t) > Battery maximum energy rate
      | than punish
  note: Battery is low and discharging
      | than punish
  note: Battery is full and charging
      | than punish
  note: Battery Power -----> Battery Capacity (kWh) -----> Battery SOC Battery Charge Power
      | Battery Discharge Power
  note: Battery Capacity
  note: SOC
      | Discharging at low battery SOC
  note: SOC
      | Battery Overcharging
  note: Charging power
      | Battery Overcharging
  note: Discharging power
      | Battery Overdischarging
  battery_capacity : Inport
  battery_capacity_upper_limit : Inport  Port=2
  battery_SOC : Inport  Port=3
  battery_SOC_lower_limit : Inport  Port=4
  battery_SOC_upper_limit : Inport  Port=5
  battery_charging_power : Inport  Port=6
  battery_charging_power_upper_limit : Inport  Port=7
  battery_discharging_power : Inport  Port=8
  battery_discharging_power_upper_limit : Inport  Port=9
  Abs : Abs  SaturateOnIntegerOverflow=off
  Battery capacity Utilization overlimit Battery charging / discharging overcurrent : RelationalOperator  Operator=>  OutDataTypeStr=boolean  RndMeth=Simplest  InputSameDT=off
  Battery full charged : RelationalOperator  Operator=>  OutDataTypeStr=boolean  RndMeth=Simplest  InputSameDT=off
  Battery low : RelationalOperator  Operator=<=  OutDataTypeStr=boolean  RndMeth=Simplest  InputSameDT=off
  Charging at Full battery SOC : Logic  IconShape=distinctive  AllPortsSameDT=off  OutDataTypeStr=boolean
  NOT{,1..4} (5 alike) : Logic  Operator=NOT  IconShape=distinctive  AllPortsSameDT=off  OutDataTypeStr=boolean
  Overcharging Rate battery SOC : RelationalOperator  Operator=>  OutDataTypeStr=boolean  RndMeth=Simplest  InputSameDT=off
  Overdischarging Rate battery SOC : RelationalOperator  Operator=>  OutDataTypeStr=boolean  RndMeth=Simplest  InputSameDT=off
  charging : simulink/Logic and Bit Operations/Compare To Zero  relop=>  OutDataTypeStr=boolean
  discharging : simulink/Logic and Bit Operations/Compare To Zero  relop=>  OutDataTypeStr=boolean
  discharging at low battery SOC : Logic  IconShape=distinctive  AllPortsSameDT=off  OutDataTypeStr=boolean
  Battery capacity Reward : Outport
  Battery capacity Punishment : Outport  Port=2
  Discharging at Low Battery SOC Reward : Outport  Port=3
  Discharging at Low Battery SOC Punish : Outport  Port=4
  Overcharging Reward : Outport  Port=5
  Overcharging Punish : Outport  Port=6
  Overcharging Rate Reward : Outport  Port=7
  Overcharging Rate Punish : Outport  Port=8
  Overdischarging Rate Reward : Outport  Port=9
  Overdischarging Rate Punish : Outport  Port=10
  wires:
  Battery low/1 -> discharging at low battery SOC/1
  discharging/1 -> discharging at low battery SOC/2
  battery_charging_power/1 -> Overcharging Rate battery SOC/1, charging/1
  charging/1 -> Charging at Full battery SOC/2
  discharging at low battery SOC/1 -> NOT1/1, Discharging at Low Battery SOC Punish/1  "Discharging at  Low Battery  SOC Punish"
  Battery capacity Utilization overlimit Battery charging / discharging overcurrent/1 -> NOT/1, Battery capacity Punishment/1  "Battery capacity  Punishment"
  Abs/1 -> Battery capacity Utilization overlimit Battery charging / discharging overcurrent/1
  Battery full charged/1 -> Charging at Full battery SOC/1  "s"
  battery_SOC/1 -> Battery low/1, Battery full charged/1
  Overdischarging Rate battery SOC/1 -> NOT4/1, Overdischarging Rate Punish/1  "Overdischarging  Rate Punish"
  Charging at Full battery SOC/1 -> NOT2/1, Overcharging Punish/1  "Overcharging  Punish"
  battery_SOC_upper_limit/1 -> Battery full charged/2
  battery_capacity_upper_limit/1 -> Battery capacity Utilization overlimit Battery charging / discharging overcurrent/2
  battery_capacity/1 -> Abs/1
  battery_charging_power_upper_limit/1 -> Overcharging Rate battery SOC/2
  Overcharging Rate battery SOC/1 -> NOT3/1, Overcharging Rate Punish/1  "Overcharging  Rate Punish"
  battery_SOC_lower_limit/1 -> Battery low/2
  battery_discharging_power/1 -> Overdischarging Rate battery SOC/1, discharging/1
  battery_discharging_power_upper_limit/1 -> Overdischarging Rate battery SOC/2
  NOT/1 -> Battery capacity Reward/1
  NOT1/1 -> Discharging at Low Battery SOC Reward/1
  NOT2/1 -> Overcharging Reward/1
  NOT3/1 -> Overcharging Rate Reward/1
  NOT4/1 -> Overdischarging Rate Reward/1
